simulink model "fluid"  (R2020a)
settings: Solver=VariableStepAuto  StartTime=0.0  StopTime=800.0  MaxStep=1  RelTol=1e-3
PreLoadFcn:
  | r1 = 40;
  | r2 = 40;
  | r3 = 40;
  | a1 = 2;
  | a2 = 3;
InitFcn:
  | r1 = 40;
  | r2 = 40;
  | r3 = 40;
  | a1 = 2;
  | a2 = 3;
settings Model: Creator=muham  LastModifiedBy=muham

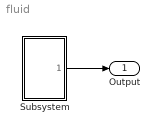
== system fluid ==
  Subsystem : Subsystem
  Output : Outport
  wires:
  Subsystem/1(Output) -> Output/1

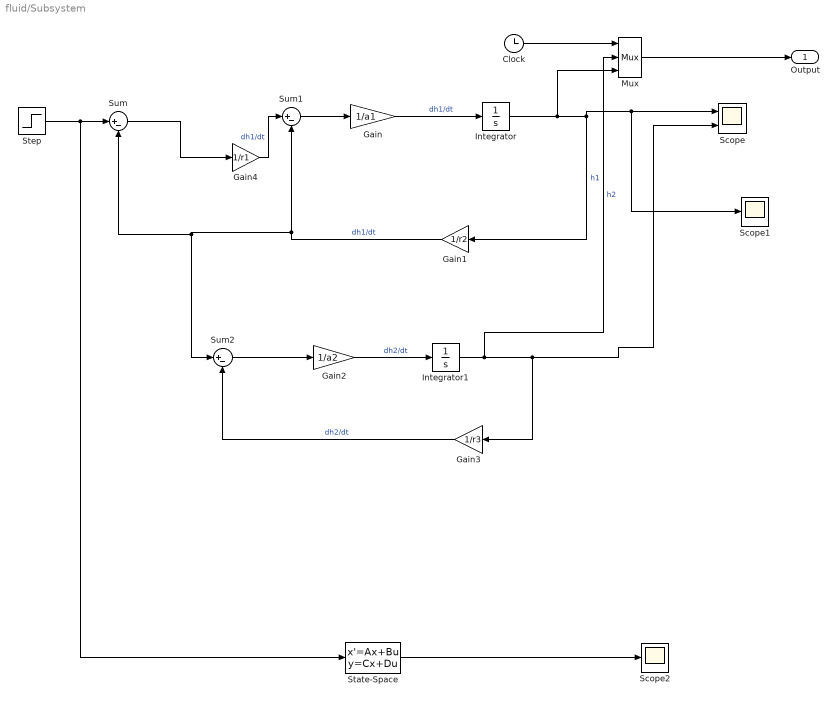
== system fluid/Subsystem ==
  Clock : Clock
  Gain : Gain  Gain=1/a1
  Gain1 : Gain  Gain=1/r2
  Gain2 : Gain  Gain=1/a2
  Gain3 : Gain  Gain=1/r3
  Gain4 : Gain  Gain=1/r1
  Integrator : Integrator  InitialCondition=1
  Integrator1 : Integrator
  Mux : Mux  Inputs=3
  Scope : Scope  NumInputPorts=2
  Scope1 : Scope
  Scope2 : Scope
  State-Space : StateSpace  A=[-1/(r1*a1)-(1/(r2*a2)),0;1/(r2*a2),-1/(r3*a2)]  B=[1/(r1*a1);0]  C=[1 0;0 1]  D=[0;0]  InitialCondition=0
  Step : Step  After=12  SampleTime=0
  Sum : Sum  Inputs=|+-
  Sum1 : Sum  Inputs=|+-
  Sum2 : Sum  Inputs=|+-
  Output : Outport
  wires:
  Gain4/1 -> Sum1/1  "dh1/dt"
  Integrator/1 -> Mux/3, Gain1/1, Scope1/1, Scope/1  "h1"
  Sum2/1 -> Gain2/1
  Gain1/1 -> Sum/2, Sum2/1, Sum1/2  "dh1/dt"
  Step/1 -> State-Space/1, Sum/1
  Gain2/1 -> Integrator1/1  "dh2/dt"
  State-Space/1 -> Scope2/1
  Integrator1/1 -> Mux/2, Scope/2, Gain3/1  "h2"
  Sum/1 -> Gain4/1
  Sum1/1 -> Gain/1
  Clock/1 -> Mux/1
  Gain3/1 -> Sum2/2  "dh2/dt"
  Mux/1 -> Output/1
  Gain/1 -> Integrator/1  "dh1/dt"
